simulink model "Hybrid_automata"  (R2017b)
settings: Solver=FixedStepAuto  StartTime=0.0  StopTime=10.0  RelTol=1e-3  EnableMultiTasking=on
model workspace (MAT data in the model file):
  Param = Simulink.Parameter
  Param.DataType = 'auto'
  Param.Dimensions = [0 0]
values from neighbouring files (symbols this model uses):
  K = acker(s1z.a, s1z.b, [0.2225 0.9743 0.987 0.987])    [model.m]
  K_PWM = 8.087    [model.m]
  l = 0.125    [model.m]
  R = 0.027    [model.m]
  Ts = 0.0033    [model.m]
undefined symbols (not defined in the file or in its folder): DiscIntNeverNeededParam
libraries: legoev3lib x6, simulink x3
settings Model: ExtModeTrigDuration=2  Creator=USER  LastModifiedBy=USER
settings SolverCC: PositivePriorityOrder=on
settings OptimizationCC: PassReuseOutputArgsAs=Individual arguments  MaxStackSize=64
settings DebuggingCC: UnderspecifiedInitializationDetection=Classic  MergeDetectMultiDrivingBlocksExec=none  ParameterTunabilityLossMsg=error
settings HardwareCC: ProdBitPerPointer=32  ProdBitPerSizeT=32  ProdBitPerPtrDiffT=32  ProdLargestAtomicInteger=Long  ProdWordSize=32  ProdHWDeviceType=ARM Compatible->ARM 9
settings SFSimCC: MATLABDynamicMemAlloc=off
settings RTWCC: SystemTargetFile=ert.tlc  HardwareBoard=LEGO MINDSTORMS EV3  TemplateMakefile=ert_default_tmf  GenerateReport=on  Toolchain=Sourcery G++ Lite v2009q3  IncludeHyperlinkInReport=on  LaunchReport=on  GenerateTraceInfo=on  GenerateTraceReport=on  GenerateTraceReportSl=on  GenerateTraceReportSf=on  GenerateTraceReportEml=on
settings CodeAppCC: ForceParamTrailComments=on  IgnoreCustomStorageClasses=off  OperatorAnnotations=on  SimulinkDataObjDesc=on  SFDataObjDesc=on  InsertBlockDesc=on
settings ERTTargetCC: SupportContinuousTime=on  SupportVariableSizeSignals=on

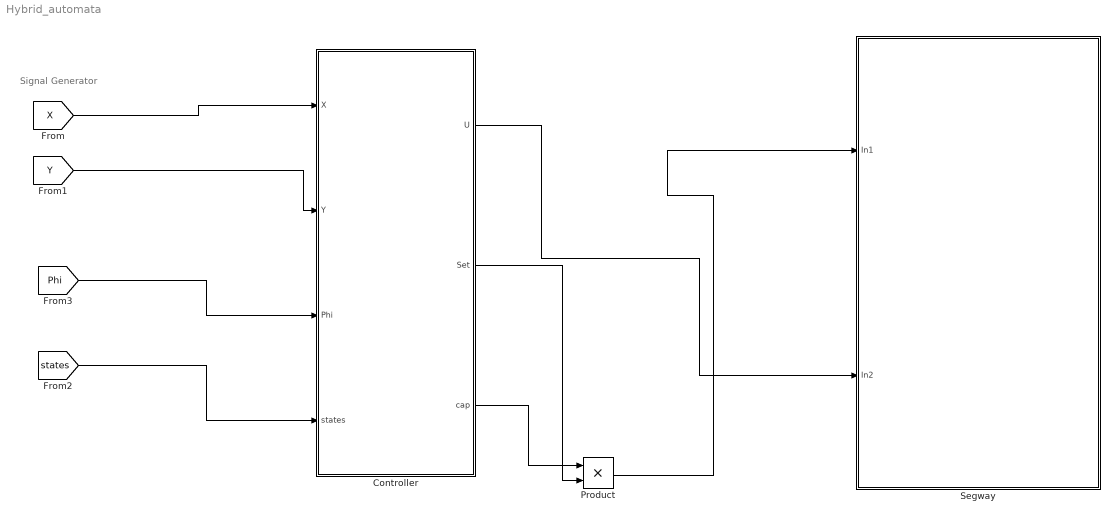
== system Hybrid_automata ==
  note: Signal Generator
  Controller : Stateflow chart  TreatAsAtomicUnit=on
  Product : Product
  "Segway " : Subsystem
      mask Display: image('C:\Users\USER\Desktop\presentation 1\assemblé complet.png');
  wires:
  [X] -> Controller/1(X)
  [Y] -> Controller/2(Y)
  [states] -> Controller/4(states)
  [Phi] -> Controller/3(Phi)
  Controller/2(Set) -> Product/2
  Controller/3(cap) -> Product/1
  Product/1 -> "Segway "/1(In1)
  Controller/1(U) -> "Segway "/2(In2)

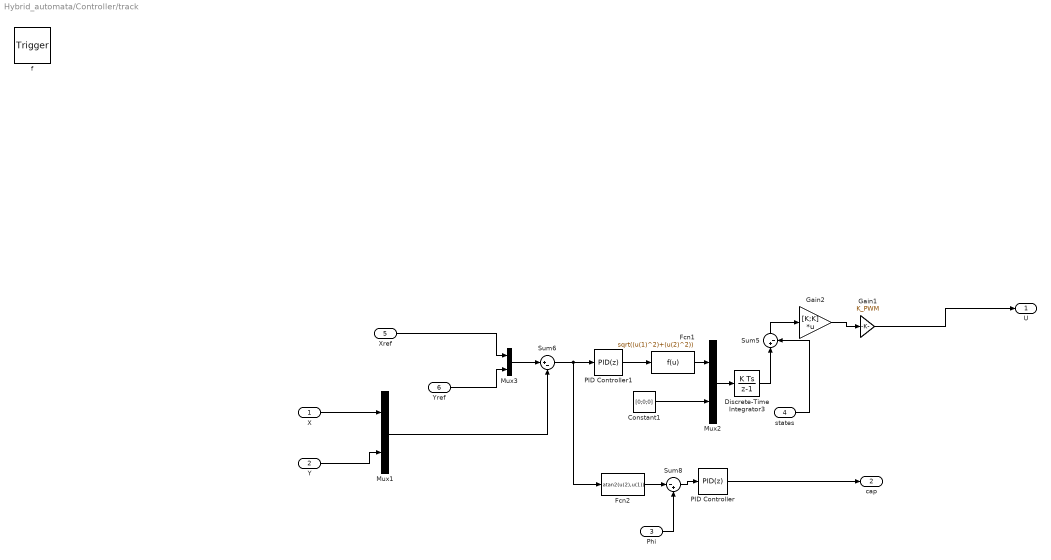
== system Hybrid_automata/Controller/track ==
  X : Inport  OutDataTypeStr=double  PortDimensions=1
  Y : Inport  Port=2  OutDataTypeStr=double  PortDimensions=1
  Phi : Inport  Port=3  OutDataTypeStr=double  PortDimensions=1
  states : Inport  Port=4  OutMin=[4]  OutMax=[4]  OutDataTypeStr=double  PortDimensions=4
  Xref : Inport  Port=5  OutDataTypeStr=double  PortDimensions=1
  Yref : Inport  Port=6  OutDataTypeStr=double  PortDimensions=1
  f : TriggerPort  TriggerType=function-call  VariantControl=(inherit)
      settings: CopyFcn=Stateflow.SLINSF.SimulinkMan.removeBlockPreDeleteFcn  PreDeleteFcn=Stateflow.SLINSF.SimulinkMan.unsafePredeleteFcn
  Constant1 : Constant  Value=[0;0;0]
  Discrete-Time Integrator3 : DiscreteIntegrator  SampleTime=-1  ICPrevOutput=DiscIntNeverNeededParam  ICPrevScaledInput=DiscIntNeverNeededParam
  Fcn1 : Fcn  Expr=sqrt((u(1)^2)+(u(2)^2))
  Fcn2 : Fcn  Expr=atan2(u(2),u(1))
  Gain1 : Gain  Gain=K_PWM
  Gain2 : Gain  Gain=[K;K]  Multiplication=Matrix(K*u)
  Mux1 : Mux  Inputs=2
  Mux2 : Mux  Inputs=2
  Mux3 : Mux  Inputs=2
  PID Controller : simulink/Continuous/PID Controller  Controller=PID  TimeDomain=Discrete-time  SampleTime=-1  IntegratorMethod=Forward Euler  FilterMethod=Forward Euler  Form=Parallel  UseFilter=on  ControllerParametersSource=internal  P=4  I=0  D=0.8  N=100  InitialConditionSource=internal  InitialConditionForIntegrator=0  InitialConditionForFilter=0  ExternalReset=none  LimitOutput=off  UpperSaturationLimit=inf  LowerSaturationLimit=-inf  LinearizeAsGain=on  AntiWindupMode=none  Kb=1  TrackingMode=off  Kt=1  PParamMin=[]  PParamMax=[]  IParamMin=[]  IParamMax=[]  DParamMin=[]  DParamMax=[]  NParamMin=[]  NParamMax=[]  KbParamMin=[]  KbParamMax=[]  KtParamMin=[]  KtParamMax=[]  POutMin=[]  POutMax=[]  IOutMin=[]  IOutMax=[]  DOutMin=[]  DOutMax=[]  NOutMin=[]  NOutMax=[]  KbOutMin=[]  KbOutMax=[]  KtOutMin=[]  KtOutMax=[]  IntegratorOutMin=[]  IntegratorOutMax=[]  FilterOutMin=[]  FilterOutMax=[]  SumOutMin=[]  SumOutMax=[]  SumI1OutMin=[]  SumI1OutMax=[]  SumI2OutMin=[]  SumI2OutMax=[]  SumI3OutMin=[]  SumI3OutMax=[]  SumDOutMin=[]  SumDOutMax=[]  SaturationOutMin=[]  SaturationOutMax=[]  IntegratorContinuousStateAttributes=''  IntegratorStateMustResolveToSignalObject=off  IntegratorRTWStateStorageClass=Auto  FilterContinuousStateAttributes=''  FilterStateMustResolveToSignalObject=off  FilterRTWStateStorageClass=Auto  DifferentiatorICPrevScaledInput=0  DifferentiatorOutMin=[]  DifferentiatorOutMax=[]  InitialConditionSetting=State (most efficient)  FilterDiffOutCoefMin=[]  FilterDiffOutCoefMax=[]  SumDenOutMin=[]  SumDenOutMax=[]  SumNumOutMin=[]  SumNumOutMax=[]  ReciprocalOutMin=[]  ReciprocalOutMax=[]  DivideOutMin=[]  DivideOutMax=[]  TunerSelectOption=Transfer Function Based (PID Tuner App)
  PID Controller1 : simulink/Continuous/PID Controller  Controller=PID  TimeDomain=Discrete-time  SampleTime=-1  IntegratorMethod=Forward Euler  FilterMethod=Forward Euler  Form=Parallel  UseFilter=on  ControllerParametersSource=internal  P=1  I=0.025  D=0.105  N=100  InitialConditionSource=internal  InitialConditionForIntegrator=0  InitialConditionForFilter=0  ExternalReset=none  LimitOutput=off  UpperSaturationLimit=inf  LowerSaturationLimit=-inf  LinearizeAsGain=on  AntiWindupMode=none  Kb=1  TrackingMode=off  Kt=1  PParamMin=[]  PParamMax=[]  IParamMin=[]  IParamMax=[]  DParamMin=[]  DParamMax=[]  NParamMin=[]  NParamMax=[]  KbParamMin=[]  KbParamMax=[]  KtParamMin=[]  KtParamMax=[]  POutMin=[]  POutMax=[]  IOutMin=[]  IOutMax=[]  DOutMin=[]  DOutMax=[]  NOutMin=[]  NOutMax=[]  KbOutMin=[]  KbOutMax=[]  KtOutMin=[]  KtOutMax=[]  IntegratorOutMin=[]  IntegratorOutMax=[]  FilterOutMin=[]  FilterOutMax=[]  SumOutMin=[]  SumOutMax=[]  SumI1OutMin=[]  SumI1OutMax=[]  SumI2OutMin=[]  SumI2OutMax=[]  SumI3OutMin=[]  SumI3OutMax=[]  SumDOutMin=[]  SumDOutMax=[]  SaturationOutMin=[]  SaturationOutMax=[]  IntegratorContinuousStateAttributes=''  IntegratorStateMustResolveToSignalObject=off  IntegratorRTWStateStorageClass=Auto  FilterContinuousStateAttributes=''  FilterStateMustResolveToSignalObject=off  FilterRTWStateStorageClass=Auto  DifferentiatorICPrevScaledInput=0  DifferentiatorOutMin=[]  DifferentiatorOutMax=[]  InitialConditionSetting=State (most efficient)  FilterDiffOutCoefMin=[]  FilterDiffOutCoefMax=[]  SumDenOutMin=[]  SumDenOutMax=[]  SumNumOutMin=[]  SumNumOutMax=[]  ReciprocalOutMin=[]  ReciprocalOutMax=[]  DivideOutMin=[]  DivideOutMax=[]  TunerSelectOption=Transfer Function Based (PID Tuner App)
  Sum5 : Sum  Inputs=|+-
  Sum6 : Sum  Inputs=|+-
  Sum8 : Sum  Inputs=|-+
  U : Outport  InitialOutput=[0;0]
  cap : Outport  Port=2  InitialOutput=[0]
  wires:
  Y/1 -> Mux1/2
  X/1 -> Mux1/1
  Discrete-Time Integrator3/1 -> Sum5/1
  Fcn1/1 -> Mux2/1
  Phi/1 -> Sum8/2
  Xref/1 -> Mux3/1
  Sum5/1 -> Gain2/1
  Yref/1 -> Mux3/2
  Sum8/1 -> PID Controller/1
  Fcn2/1 -> Sum8/1
  Mux2/1 -> Discrete-Time Integrator3/1
  Sum6/1 -> PID Controller1/1, Fcn2/1
  Gain2/1 -> Gain1/1
  PID Controller1/1 -> Fcn1/1
  Mux1/1 -> Sum6/2
  Constant1/1 -> Mux2/2
  Mux3/1 -> Sum6/1
  Gain1/1 -> U/1
  states/1 -> Sum5/2
  PID Controller/1 -> cap/1

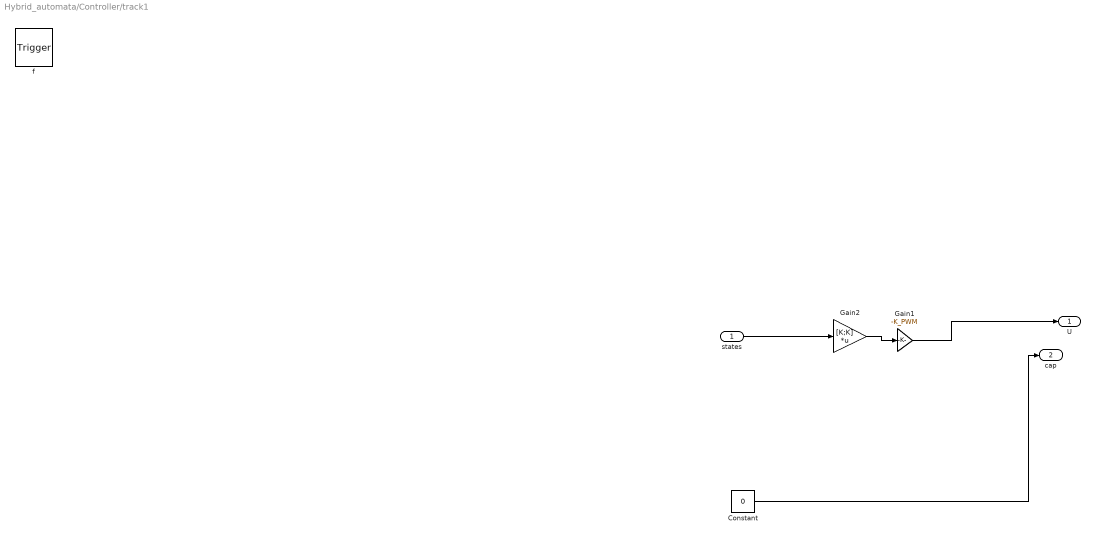
== system Hybrid_automata/Controller/track1 ==
  states : Inport  OutMin=[4]  OutMax=[4]  OutDataTypeStr=double  PortDimensions=4
  f : TriggerPort  TriggerType=function-call  VariantControl=(inherit)
      settings: CopyFcn=Stateflow.SLINSF.SimulinkMan.removeBlockPreDeleteFcn  PreDeleteFcn=Stateflow.SLINSF.SimulinkMan.unsafePredeleteFcn
  Constant : Constant  Value=0
  Gain1 : Gain  Gain=-K_PWM
  Gain2 : Gain  Gain=[K;K]  Multiplication=Matrix(K*u)
  U : Outport  InitialOutput=[0;0]
  cap : Outport  Port=2  InitialOutput=[0]
  wires:
  states/1 -> Gain2/1
  Gain2/1 -> Gain1/1
  Gain1/1 -> U/1
  Constant/1 -> cap/1

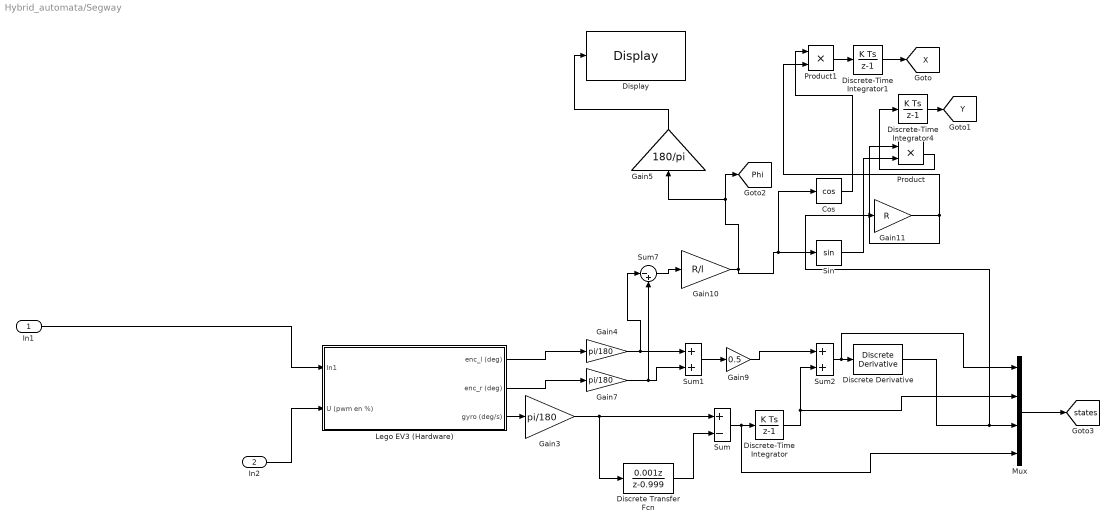
== system Hybrid_automata/Segway  ==
  In1 : Inport
  In2 : Inport  Port=2
  Cos : Trigonometry  Operator=cos
  Discrete Transfer Fcn : DiscreteTransferFcn  Numerator=[0.001 0]  Denominator=[1 -0.999]  SampleTime=Ts
  Discrete Derivative : simulink/Discrete/Discrete Derivative  gainval=1.0  ICPrevScaledInput=0.0  OutMin=[]  OutMax=[]  OutDataType=fixdt(1, 16)  OutScaling=2^-10  DoSatur=off
  Discrete-Time Integrator : DiscreteIntegrator  InitialConditionSetting=State (most efficient)  SampleTime=Ts  ICPrevOutput=DiscIntNeverNeededParam  ICPrevScaledInput=DiscIntNeverNeededParam
  Discrete-Time Integrator1 : DiscreteIntegrator  InitialConditionSetting=State (most efficient)  SampleTime=Ts  ICPrevOutput=DiscIntNeverNeededParam  ICPrevScaledInput=DiscIntNeverNeededParam
  Discrete-Time Integrator4 : DiscreteIntegrator  InitialConditionSetting=State (most efficient)  SampleTime=Ts  ICPrevOutput=DiscIntNeverNeededParam  ICPrevScaledInput=DiscIntNeverNeededParam
  Display : legoev3lib/Display  slcdLine=1  slcdFormat=Decimal
      settings: SourceProductName=Simulink Support Package for LEGO MINDSTORMS EV3 Hardware  SourceProductBaseCode=LEGOEV3
  Gain10 : Gain  Gain=R/l
  Gain11 : Gain  Gain=R
  Gain3 : Gain  Gain=pi/180
  Gain4 : Gain  Gain=pi/180
  Gain5 : Gain  Gain=180/pi
  Gain7 : Gain  Gain=pi/180
  Gain9 : Gain  Gain=0.5
  Lego EV3 (Hardware) : Subsystem
  Mux : Mux
  Product : Product
  Product1 : Product
  Sin : Trigonometry
  Sum : Sum  Inputs=+-
  Sum1 : Sum
  Sum2 : Sum
  Sum7 : Sum  Inputs=|-+
  tag scope: Phi=global, X=global, Y=global, states=global
  wires:
  Gain10/1 -> Cos/1, Sin/1, Gain5/1, [Phi]
  Discrete-Time Integrator4/1 -> [Y]
  In2/1 -> Lego EV3 (Hardware)/2(U (pwm en %))
  Product1/1 -> Discrete-Time Integrator1/1
  Discrete Transfer Fcn/1 -> Sum/2
  In1/1 -> Lego EV3 (Hardware)/1(In1)
  Gain9/1 -> Sum2/1
  Lego EV3 (Hardware)/1(enc_l (deg)) -> Gain4/1
  Lego EV3 (Hardware)/2(enc_r (deg)) -> Gain7/1
  Gain4/1 -> Sum7/1, Sum1/1
  Discrete-Time Integrator1/1 -> [X]
  Sin/1 -> Product/2
  Discrete Derivative/1 -> Gain11/1, Mux/3
  Sum7/1 -> Gain10/1
  Product/1 -> Discrete-Time Integrator4/1
  Gain5/1 -> Display/1
  Sum2/1 -> Mux/1, Discrete Derivative/1
  Sum/1 -> Mux/4, Discrete-Time Integrator/1
  Lego EV3 (Hardware)/3(gyro (deg/s)) -> Gain3/1
  Mux/1 -> [states]
  Sum1/1 -> Gain9/1
  Cos/1 -> Product1/1
  Gain3/1 -> Discrete Transfer Fcn/1, Sum/1
  Discrete-Time Integrator/1 -> Mux/2, Sum2/2
  Gain7/1 -> Sum7/2, Sum1/2
  Gain11/1 -> Product/1, Product1/2

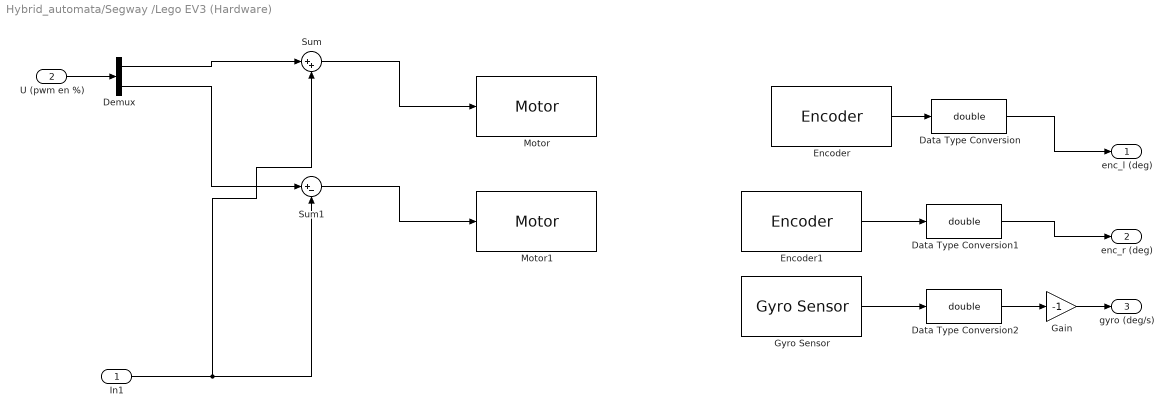
== system Hybrid_automata/Segway /Lego EV3 (Hardware) ==
  In1 : Inport
  U (pwm en %) : Inport  Port=2
  Data Type Conversion : DataTypeConversion  OutDataTypeStr=double
  Data Type Conversion1 : DataTypeConversion  OutDataTypeStr=double
  Data Type Conversion2 : DataTypeConversion  OutDataTypeStr=double
  Demux : Demux  Outputs=2
  Encoder : legoev3lib/Encoder  portNumber=D  opMode=No reset  sampleTime=Ts
      settings: SourceProductName=Simulink Support Package for LEGO MINDSTORMS EV3 Hardware  SourceProductBaseCode=LEGOEV3
  Encoder1 : legoev3lib/Encoder  portNumber=A  opMode=No reset  sampleTime=Ts
      settings: SourceProductName=Simulink Support Package for LEGO MINDSTORMS EV3 Hardware  SourceProductBaseCode=LEGOEV3
  Gain : Gain  Gain=-1
  Gyro Sensor : legoev3lib/Gyro Sensor  portNumber=3  sampleTime=Ts
      settings: SourceProductName=Simulink Support Package for LEGO MINDSTORMS EV3 Hardware  SourceProductBaseCode=LEGOEV3
  Motor : legoev3lib/Motor  sportNumber=D  sstopAction=Brake
  Motor1 : legoev3lib/Motor  sportNumber=A  sstopAction=Brake
  Sum : Sum  Inputs=|++
  Sum1 : Sum  Inputs=|+-
  enc_l (deg) : Outport  VectorParamsAs1DForOutWhenUnconnected=on
  enc_r (deg) : Outport  Port=2  VectorParamsAs1DForOutWhenUnconnected=on
  gyro (deg/s) : Outport  Port=3  VectorParamsAs1DForOutWhenUnconnected=on
  wires:
  Gyro Sensor/1 -> Data Type Conversion2/1
  Encoder1/1 -> Data Type Conversion1/1
  Encoder/1 -> Data Type Conversion/1
  Data Type Conversion/1 -> enc_l (deg)/1
  Data Type Conversion1/1 -> enc_r (deg)/1
  Data Type Conversion2/1 -> Gain/1
  Gain/1 -> gyro (deg/s)/1
  U (pwm en %)/1 -> Demux/1
  Demux/1 -> Sum/1
  Demux/2 -> Sum1/1
  Sum/1 -> Motor/1
  Sum1/1 -> Motor1/1
  In1/1 -> Sum/2, Sum1/2

== stateflow chart Hybrid_automata/Controller ==
  settings: updateMethod=DISCRETE  sampleTime=0.0033
  state GoToGoal
    entry:
    i=1;
    P=waypoints(:,i);
    Xref=P(1);
    Yref=P(2);
    %Set=0;
    Set=1;
    during:
    % [U,cap]=track1(states);
    [U,cap]= track(X,Y,Phi,states,Xref,Yref);
    V=sqrt(((Xref-X)^2)+((Yref-Y)^2));
  state Stop
    during:
    Set=0;
    [U,cap]=track1(states);
  state NextGoal [commented out]
    entry:
    P=waypoints(:,i)
    Xref=P(1);
    Yref=P(2);
    during:
    Set=1;
    [U,cap]= track(X,Y,Phi,states,Xref,Yref);
    V=sqrt(((Xref-X)^2)+((Yref-Y)^2));
    exit:
    i=i+1;
  state Track [commented out]
    during:
    [U,cap]= track(X,Y,Phi,states,Xref,Yref),Set=1;
    V=sqrt(((Xref-X)^2)+((Yref-Y)^2));
    exit:
    i=i+1;
  state [U,cap] = track1(states) [function]
  state [U,cap] = track(X,Y,Phi,states,Xref,Yref) [function]
  (default) -> GoToGoal
  Stop -> NextGoal [commented out] : [after(2,sec)]
  GoToGoal -> Stop : [V<0.1]{i=i+1;}
  NextGoal -> Stop [commented out] : [V<0.02 ]
  Stop -> Stop [commented out] : [norm(P-waypoints(:,4))==0]
  (default) -> Track [commented out] : [after(3,sec)]
  data: U function_output; states function_input double size=4; cap function_output; X function_input double size=1; Y function_input double size=1; Phi function_input double size=1; U function_output; states function_input double size=4; Xref function_input double size=1; Yref function_input double size=1; cap function_output; X input; Y input; Phi input; states input double size=[4,1] [4..4]; U output [4..4]; waypoints parameter; i local; P local; Yref local; Xref local; V local; Set output; cap output
